simulink model "mdl_VD_KinematicBicycleModel_R2023b_SLX"  (R2023b)
settings: Solver=ode4  StartTime=startTime  StopTime=endTime  FixedStep=deltaT  MaxStep=deltaT  RelTol=1e-3  EnableMultiTasking=on
values from neighbouring files (symbols this model uses):
  L = a+b    [script_test_mdl_VD_KinematicBicycleModel.m]
  U = 20    [script_test_mdl_VD_KinematicBicycleModel.m]
undefined symbols (not defined in the file or in its folder): initialStates
settings Model: Creator=snb10  LastModifiedBy=snb10
settings SolverCC: AlgebraicLoopSolver=TrustRegion
settings DataIOCC: LimitDataPoints=on  SaveFormat=Array  SignalLoggingSaveFormat=ModelDataLogs  SaveOutput=off  SignalLogging=off  DSMLogging=off  SaveTime=off  SignalLoggingName=sigsOut
settings OptimizationCC: InitFltsAndDblsToZero=on  LifeSpan=inf
settings DebuggingCC: SaveWithParameterizedLinksMsg=none  UnderspecifiedInitializationDetection=Classic  MergeDetectMultiDrivingBlocksExec=none  SignalResolutionControl=TryResolveAllWithWarning  MultiTaskDSMMsg=warning  MultiTaskCondExecSysMsg=none  FcnCallInpInsideContextMsg=warning  UnconnectedInputMsg=warning  UnconnectedOutputMsg=warning  UnconnectedLineMsg=warning  StateNameClashWarn=warning  SFUnexpectedBacktrackingDiag=warning  SFNoUnconditionalDefaultTransitionDiag=warning  SFExecutionAtInitializationDiag=none  ArithmeticOperatorsInVariantConditions=warning
settings HardwareCC: ProdBitPerPointer=32  ProdBitPerSizeT=32  ProdBitPerPtrDiffT=32  ProdLargestAtomicFloat=None  ProdIntDivRoundTo=Undefined  ProdEndianess=Unspecified  ProdWordSize=32  ProdHWDeviceType=32-bit Generic  TargetUnknown=on
settings ModelReferenceCC: EnableRefExpFcnMdlSchedulingChecks=on  PropagateSignalLabelsOutOfModel=off
settings SFSimCC: SimUseLocalCustomCode=off  CustomCodeUndefinedFunction=UseInterfaceOnly
settings RTWCC: RTWUseLocalCustomCode=off  DLArmComputeVersion=19.05
settings CodeAppCC: StateflowObjectComments=on
settings GRTTargetCC: TargetFcnLib=ansi_tfl_tmw.mat  TargetLangStandard=C89/C90 (ANSI)  CombineOutputUpdateFcns=off  GRTInterface=on
settings ConfigComp: CovMetricSettings=dw  CovSaveCumulativeToWorkspaceVar=on  CovSaveSingleToWorkspaceVar=on  CovExternalEMLEnable=off  CovBoundaryAbsTol=1.0e-5

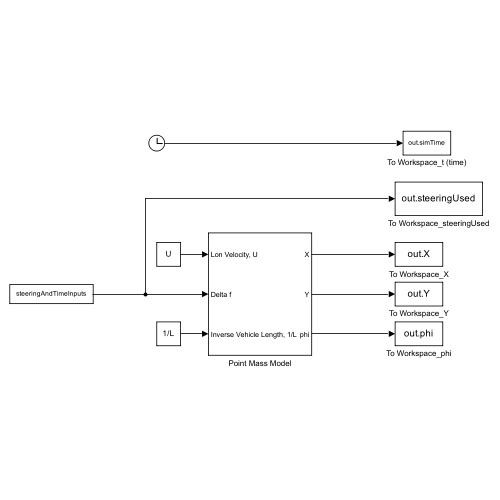
[thumbnail: Simulink's stored preview of the top-level diagram]
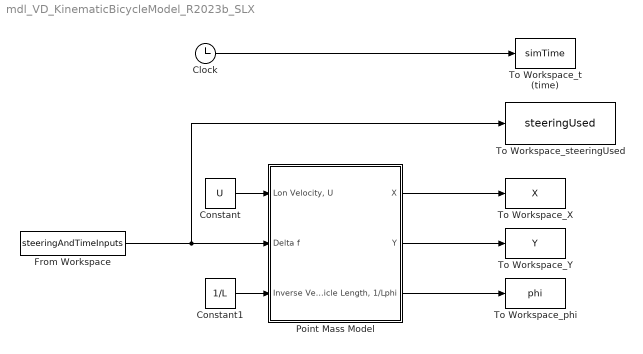
== system mdl_VD_KinematicBicycleModel_R2023b_SLX ==
  Clock : Clock
  Constant : Constant  Value=U  SampleTime=.01
  Constant1 : Constant  Value=1/L  SampleTime=.01
  From Workspace : FromWorkspace  VariableName=steeringAndTimeInputs  OutDataTypeStr=double  SampleTime=.01  OutputAfterFinalValue=Holding final value
  Point Mass Model : Subsystem
  To Workspace_X : ToWorkspace  VariableName=X  SampleTime=.01
  To Workspace_Y : ToWorkspace  VariableName=Y  SampleTime=.01
  To Workspace_phi : ToWorkspace  VariableName=phi  SampleTime=.01
  To Workspace_steeringUsed : ToWorkspace  VariableName=steeringUsed  SampleTime=.01
  To Workspace_t (time) : ToWorkspace  VariableName=simTime  SampleTime=.01
  wires:
  Clock/1 -> To Workspace_t (time)/1
  Point Mass Model/1(X) -> To Workspace_X/1
  Point Mass Model/2(Y) -> To Workspace_Y/1
  Point Mass Model/3(phi) -> To Workspace_phi/1
  From Workspace/1 -> Point Mass Model/2(Delta f), To Workspace_steeringUsed/1
  Constant/1 -> Point Mass Model/1("Lon Velocity, U")
  Constant1/1 -> Point Mass Model/3("Inverse Vehicle Length, 1/L")

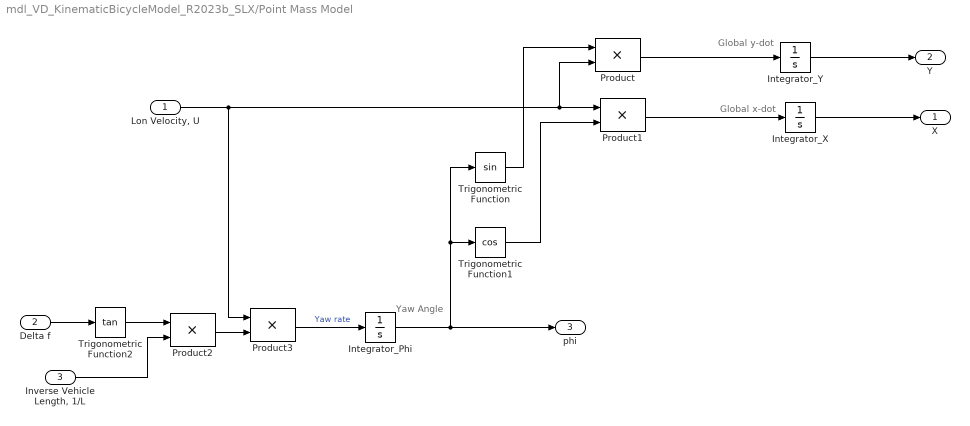
== system mdl_VD_KinematicBicycleModel_R2023b_SLX/Point Mass Model ==
  note: Global y-dot
  note: Global x-dot
  note: Yaw Angle
  "Lon Velocity, U" : Inport
  Delta f : Inport  Port=2
  "Inverse Vehicle Length, 1/L" : Inport  Port=3
  Integrator_Phi : Integrator  InitialCondition=initialStates(3)
  Integrator_X : Integrator  InitialCondition=initialStates(2)
  Integrator_Y : Integrator  InitialCondition=initialStates(1)
  Product{,1..3} (4 alike) : Product  SaturateOnIntegerOverflow=on  OutDataTypeStr=Inherit: Same as first input
  Trigonometric Function : Trigonometry
  Trigonometric Function1 : Trigonometry  Operator=cos
  Trigonometric Function2 : Trigonometry  Operator=tan
  X : Outport
  Y : Outport  Port=2
  phi : Outport  Port=3
  wires:
  Integrator_Y/1 -> Y/1
  Integrator_X/1 -> X/1
  Trigonometric Function1/1 -> Product1/2
  Product1/1 -> Integrator_X/1
  Trigonometric Function/1 -> Product/1
  Integrator_Phi/1 -> Trigonometric Function/1, Trigonometric Function1/1, phi/1
  Product/1 -> Integrator_Y/1
  Delta f/1 -> Trigonometric Function2/1
  Trigonometric Function2/1 -> Product2/1
  "Inverse Vehicle Length, 1/L"/1 -> Product2/2
  Product2/1 -> Product3/2
  "Lon Velocity, U"/1 -> Product/2, Product1/1, Product3/1
  Product3/1 -> Integrator_Phi/1  "Yaw rate"
